simulink model "Q4sim"  (R2018a)
settings: Solver=VariableStepAuto  StartTime=0.0  StopTime=10.0  RelTol=1e-3
values from neighbouring files (symbols this model uses):
  A = [0 1 0 0 ;0 -2.2626 -0.3962 0.0082; 0 0 0 1;0 3.5649 16.0655 -0.3324]    [Q1.m]    (also in Q2.m; Q3.m; Q4.m)
  B = [0; 0.2263; 0; -0.3565]    [Q1.m]    (also in Q2.m; Q3.m; Q4.m)
  F = A_ee-L*C_s*A_se    [Q4.m]
  GG = (A_es-L*C_s*A_ss)*inv(C_s)+F*L    [Q4.m]
  H = B_e-L*C_s*B_s    [Q4.m]
  K = acker(Abar,Bbar,[-1 -2 -3 -4 -5])    [Q2.m]    (also in Q3.m = acker(A,B,[-1 -2 -3 -4]); Q4.m = acker(A,B,[-1 -2 -3 -4]))
  L = acker(AA,BB(:,1),[-1 -2 -3 -4])'    [Q3.m]    (also in Q4.m = acker(A_ee',(C_s*A_se)',[-2 -3 -4])')
settings Model: Creator=Siavash  LastModifiedBy=Siavash

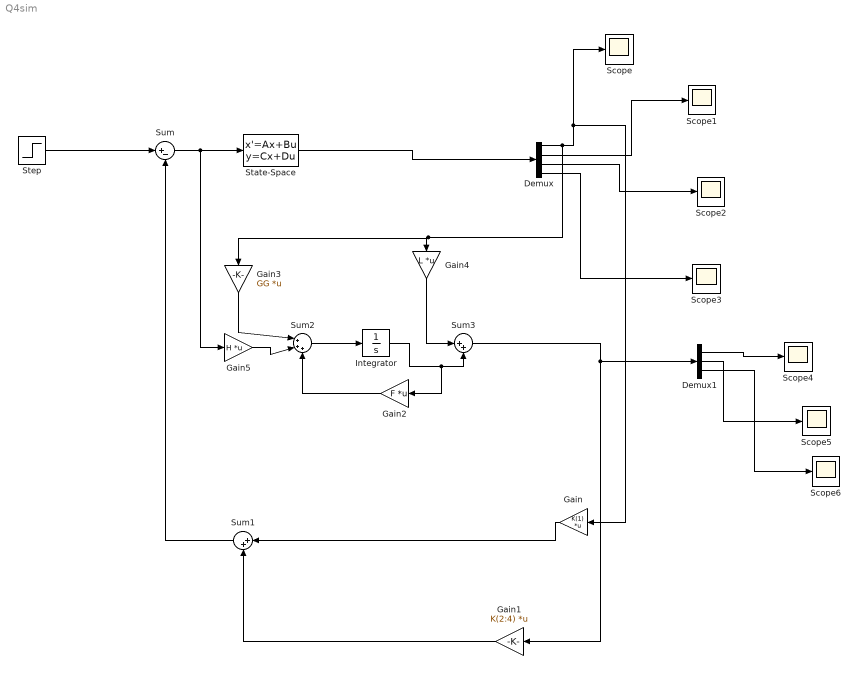
== system Q4sim ==
  Demux : Demux
  Demux1 : Demux  Outputs=3
  Gain : Gain  Gain=K(1)  Multiplication=Matrix(K*u)
  Gain1 : Gain  Gain=K(2:4)  Multiplication=Matrix(K*u)
  Gain2 : Gain  Gain=F  Multiplication=Matrix(K*u)
  Gain3 : Gain  Gain=GG  Multiplication=Matrix(K*u)
  Gain4 : Gain  Gain=L  Multiplication=Matrix(K*u)
  Gain5 : Gain  Gain=H  Multiplication=Matrix(K*u)
  Integrator : Integrator
  Scope{,1..6} (7 alike) : Scope
  State-Space : StateSpace  A=A  B=B  C=eye(4,4)  D=[0 0 0 0]'  InitialCondition=0
  Step : Step  Time=0  SampleTime=0
  Sum : Sum  Inputs=|+-
  Sum1 : Sum  Inputs=|++
  Sum2 : Sum  Inputs=|+++
  Sum3 : Sum  Inputs=|++
  wires:
  Step/1 -> Sum/1
  Sum/1 -> Gain5/1, State-Space/1
  State-Space/1 -> Demux/1
  Demux/1 -> Gain3/1, Gain4/1, Gain/1, Scope/1
  Demux/2 -> Scope1/1
  Demux/3 -> Scope2/1
  Demux/4 -> Scope3/1
  Gain/1 -> Sum1/1
  Gain1/1 -> Sum1/2
  Sum1/1 -> Sum/2
  Sum2/1 -> Integrator/1
  Gain3/1 -> Sum2/1
  Gain5/1 -> Sum2/2
  Gain2/1 -> Sum2/3
  Gain4/1 -> Sum3/1
  Integrator/1 -> Gain2/1, Sum3/2
  Sum3/1 -> Demux1/1, Gain1/1
  Demux1/1 -> Scope4/1
  Demux1/2 -> Scope5/1
  Demux1/3 -> Scope6/1
